simulink model "lab_7_task_1_simulink"  (R2025b)
settings: Solver=VariableStepAuto  StartTime=0.0  StopTime=10.0  RelTol=1e-3
values from neighbouring files (symbols this model uses):
  a = 300    [lab_7_task_1.m]    (also in lab_7_task_2.m = 7093; lab_7_task_3.m = 7093; lab_7_task_4.m = 7093; project_review.m = 7093)
  A_BN0 = eye(3)    [lab_7_task_1.m]    (also in lab_7_task_3.m; lab_7_task_4.m; project_review.m)
  e = 0    [lab_7_task_1.m]    (also in lab_7_task_2.m = 0.5; lab_7_task_3.m = 0.00277; lab_7_task_4.m = 0.00277; project_review.m = 0.00277)
  inc = 0    [lab_7_task_1.m]    (also in lab_7_task_2.m = deg2rad(98.27); lab_7_task_3.m = deg2rad(98.27); lab_7_task_4.m = deg2rad(98.27); project_review.m = deg2rad(20))
  n = sqrt(G*M_e/R^3)    [lab_6_task_1.m]    (also in lab_6_task_2.m; lab_7_task_1.m = sqrt(mu_E/(a^3)); lab_7_task_2.m = sqrt(mu_E/(a^3)); lab_7_task_3.m = sqrt(mu/(a^3)))
  TA0 = 0    [lab_7_task_1.m]    (also in lab_7_task_2.m = deg2rad(0); lab_7_task_3.m = deg2rad(0); lab_7_task_4.m = deg2rad(0); project_review.m = deg2rad(0))
libraries: dynamics x1
settings Model: Creator=nicol  LastModifiedBy=nicol

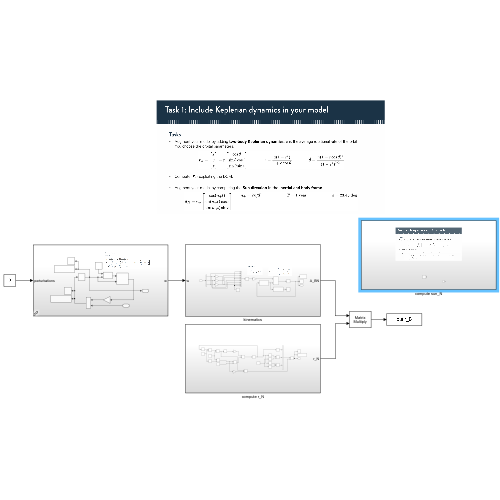
[thumbnail: Simulink's stored preview of the top-level diagram]
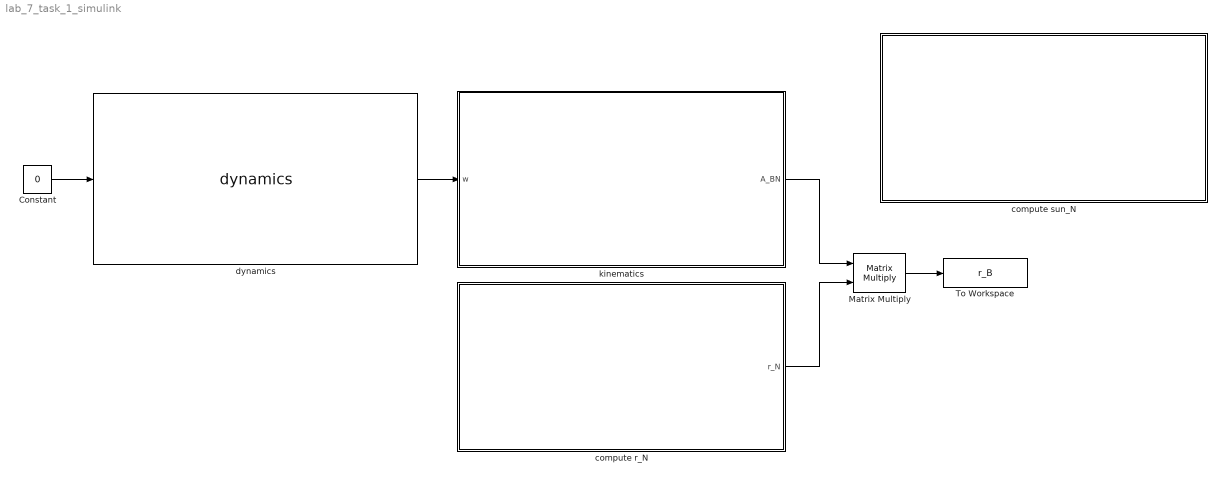
== system lab_7_task_1_simulink ==
  Constant : Constant  Value=0
  Matrix Multiply : Product  Multiplication=Matrix(*)
  To Workspace : ToWorkspace  VariableName=r_B  SaveFormat=Timeseries  SampleTime=-1
  compute r_N : Subsystem
  compute sun_N : Subsystem
  dynamics : dynamics/dynamics  SystemSampleTime=-1  VariantActivationTime=update diagram  EmptyChoice=off  PassThrough=off  PassThroughVariantControl=(default)  EmptyChoiceVariantControl=(default)  AllowFlexibleInterface=on  Latency=0  AutoFrameSizeCalculation=off
  kinematics : Subsystem
  wires:
  dynamics/1 -> kinematics/1(w)
  Constant/1 -> dynamics/1
  kinematics/1(A_BN) -> Matrix Multiply/1
  compute r_N/1(r_N) -> Matrix Multiply/2
  Matrix Multiply/1 -> To Workspace/1

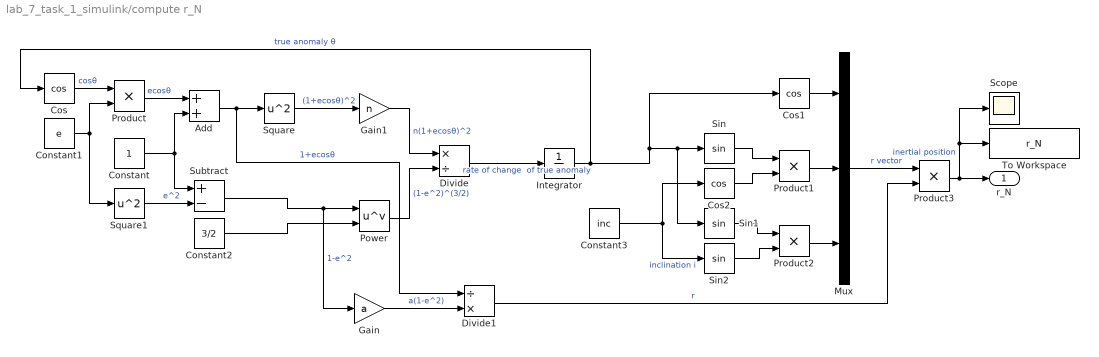
== system lab_7_task_1_simulink/compute r_N ==
  Add : Sum
  Constant : Constant
  Constant1 : Constant  Value=e
  Constant2 : Constant  Value=3/2
  Constant3 : Constant  Value=inc
  Cos : Trigonometry  Operator=cos
  Cos1 : Trigonometry  Operator=cos
  Cos2 : Trigonometry  Operator=cos
  Divide : Product  Inputs=*/
  Divide1 : Product  Inputs=/*
  Gain : Gain  Gain=a
  Gain1 : Gain  Gain=n
  Integrator : Integrator  InitialCondition=TA0
  Mux : Mux  Inputs=3
  Power : Math  Operator=pow
  Product{,1..3} (4 alike) : Product
  Scope : Scope
      settings: ActiveDisplayYMinimum=-1  ActiveDisplayYMaximum=1  DataLoggingVariableName=ScopeData3
  Sin : Trigonometry
  Sin1 : Trigonometry
  Sin2 : Trigonometry
  Square : Math  Operator=square
  Square1 : Math  Operator=square
  Subtract : Sum  Inputs=+-
  To Workspace : ToWorkspace  VariableName=r_N  SaveFormat=Timeseries  SampleTime=-1
  r_N : Outport
  wires:
  Integrator/1 -> Sin1/1, Sin/1, Cos1/1, Cos/1  "true anomaly θ"
  Add/1 -> Divide1/1, Square/1  "1+ecosθ"
  Square/1 -> Gain1/1  "(1+ecosθ)^2"
  Gain1/1 -> Divide/1  "n(1+ecosθ)^2"
  Sin1/1 -> Product2/1
  Constant/1 -> Subtract/1, Add/2
  Subtract/1 -> Gain/1, Power/1  "1-e^2"
  Product3/1 -> r_N/1, To Workspace/1, Scope/1  "inertial position"
  Constant3/1 -> Cos2/1, Sin2/1  "inclination i"
  Gain/1 -> Divide1/2  "a(1-e^2)"
  Constant2/1 -> Power/2
  Sin2/1 -> Product2/2
  Cos/1 -> Product/1  "cosθ"
  Constant1/1 -> Square1/1, Product/2
  Product/1 -> Add/1  "ecosθ"
  Product2/1 -> Mux/3
  Square1/1 -> Subtract/2  "e^2"
  Divide1/1 -> Product3/2  "r"
  Cos1/1 -> Mux/1
  Mux/1 -> Product3/1  "r vector"
  Power/1 -> Divide/2  "(1-e^2)^(3/2)"
  Product1/1 -> Mux/2
  Divide/1 -> Integrator/1  "rate of change  of true anomaly"
  Sin/1 -> Product1/1
  Cos2/1 -> Product1/2

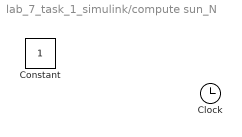
== system lab_7_task_1_simulink/compute sun_N ==
  Clock : Clock
  Constant : Constant

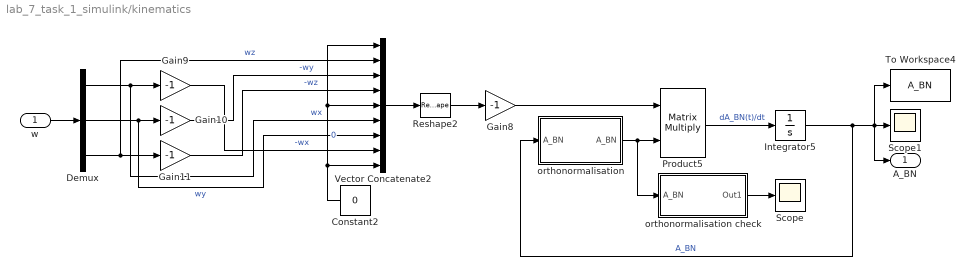
== system lab_7_task_1_simulink/kinematics ==
  w : Inport
  Constant2 : Constant  Value=0
  Demux : Demux  Outputs=3
  Gain{8..11} (4 alike) : Gain  Gain=-1
  Integrator5 : Integrator  InitialCondition=A_BN0
  Product5 : Product  Multiplication=Matrix(*)
  Reshape2 : Reshape  OutputDimensionality=Customize  OutputDimensions=[3,3]
  Scope : Scope
      settings: ActiveDisplayYMinimum=-1  ActiveDisplayYMaximum=1
  Scope1 : Scope
      settings: ActiveDisplayYMinimum=-1.2499999998899596  ActiveDisplayYMaximum=1.2499999999877733
  To Workspace4 : ToWorkspace  VariableName=A_BN  SaveFormat=Timeseries  SampleTime=-1
  Vector Concatenate2 : Concatenate  NumInputs=9
  orthonormalisation : Subsystem
  orthonormalisation check : Subsystem
  A_BN : Outport
  wires:
  Product5/1 -> Integrator5/1  "dA_BN(t)/dt"
  Gain11/1 -> Vector Concatenate2/4  "-wz"
  Integrator5/1 -> A_BN/1, To Workspace4/1, Scope1/1, orthonormalisation/1(A_BN)  "A_BN"
  Gain8/1 -> Product5/1
  Demux/1 -> Vector Concatenate2/6, Gain9/1  "wx"
  Reshape2/1 -> Gain8/1
  Gain10/1 -> Vector Concatenate2/3  "-wy"
  Demux/2 -> Vector Concatenate2/7, Gain10/1  "wy"
  Vector Concatenate2/1 -> Reshape2/1
  Demux/3 -> Vector Concatenate2/2, Gain11/1  "wz"
  Constant2/1 -> Vector Concatenate2/1, Vector Concatenate2/5, Vector Concatenate2/9  "0"
  Gain9/1 -> Vector Concatenate2/8  "-wx"
  w/1 -> Demux/1
  orthonormalisation/1(" A_BN") -> Product5/2, orthonormalisation check/1(A_BN)
  orthonormalisation check/1(Out1) -> Scope/1

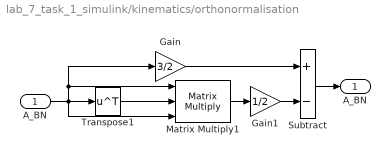
== system lab_7_task_1_simulink/kinematics/orthonormalisation ==
  A_BN : Inport
  Gain : Gain  Gain=3/2
  Gain1 : Gain  Gain=1/2
  Matrix Multiply1 : Product  Inputs=3  Multiplication=Matrix(*)
  Subtract : Sum  Inputs=+-
  Transpose1 : Math  Operator=transpose
  " A_BN" : Outport
  wires:
  Gain/1 -> Subtract/1
  Transpose1/1 -> Matrix Multiply1/2
  Matrix Multiply1/1 -> Gain1/1
  Gain1/1 -> Subtract/2
  Subtract/1 -> " A_BN"/1
  A_BN/1 -> Matrix Multiply1/1, Gain/1, Transpose1/1, Matrix Multiply1/3

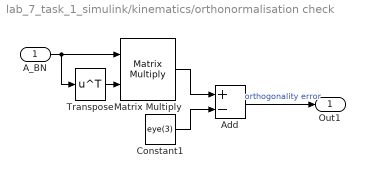
== system lab_7_task_1_simulink/kinematics/orthonormalisation check ==
  A_BN : Inport
  Add : Sum  Inputs=+-
  Constant1 : Constant  Value=eye(3)
  Matrix Multiply : Product  Multiplication=Matrix(*)
  Transpose : Math  Operator=transpose
  Out1 : Outport
  wires:
  Transpose/1 -> Matrix Multiply/2
  A_BN/1 -> Matrix Multiply/1, Transpose/1
  Add/1 -> Out1/1  "orthogonality error"
  Constant1/1 -> Add/2
  Matrix Multiply/1 -> Add/1
